simulink model "sampleModel187"  (R2021b)
settings: Solver=VariableStepAuto  StartTime=0.0  StopTime=10.0  RelTol=1e-3
undefined symbols (not defined in the file or in its folder): DiscIntNeverNeededParam, Newton, Raphson
libraries: simulink x10, slpidlib x1
settings Model: Creator=user  LastModifiedBy=user

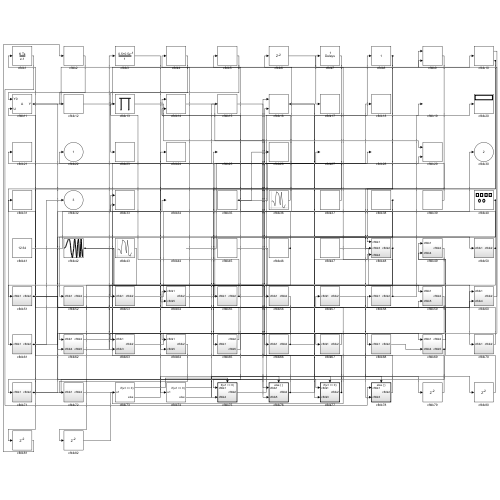
[thumbnail: Simulink's stored preview of the top-level diagram]
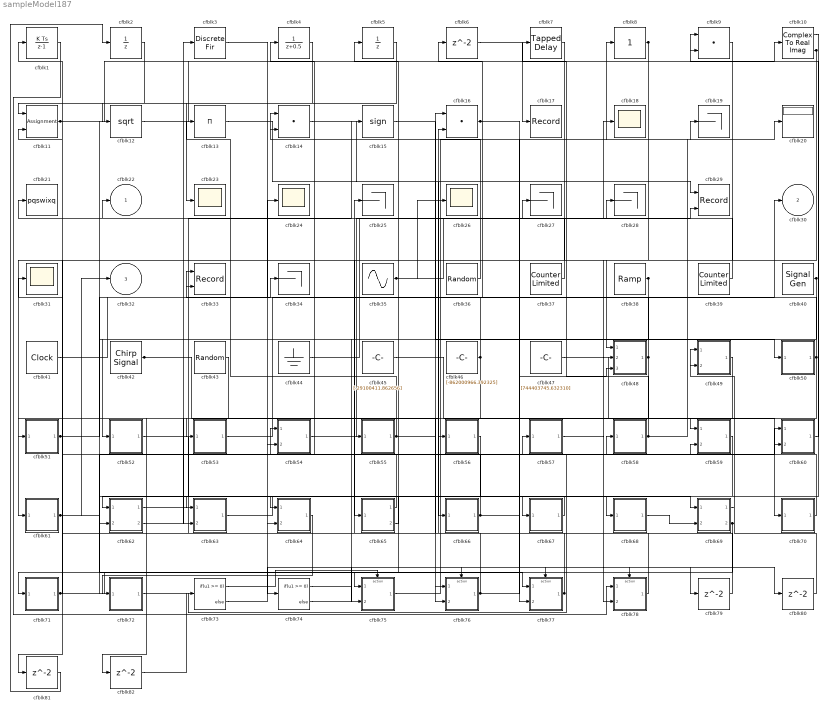
== system sampleModel187 ==
  cfblk1 : DiscreteIntegrator  ICPrevOutput=DiscIntNeverNeededParam  ICPrevScaledInput=DiscIntNeverNeededParam
  cfblk10 : ComplexToRealImag
  cfblk11 : Assignment  DiagnosticForDimensions=Warning  IndexOptions=Index vector (dialog)  Indices=1  OutputSizes=1
  cfblk12 : Sqrt  SaturateOnIntegerOverflow=on
  cfblk13 : Product  Inputs=*
  cfblk14 : DotProduct  InputSameDT=on  OutDataTypeStr=Inherit: Inherit via internal rule
  cfblk15 : Signum
  cfblk16 : DotProduct  InputSameDT=on  OutDataTypeStr=Inherit: Inherit via internal rule
  cfblk17 : Record  FileSettingsInternal="{\"entries\":[{\"content\":{\"excelSettings\":{\"content\":{},\"type\":\"Streamout.ExcelSettings\"}},\"type\":\"Streamout.FileSettingStorage\",\"uuid\":\"fc1a8ae5-f9e8-4fe5-bdf4-1e206a54b291\"}],\"packageUris\":[\"http://schema.mathworks.com/mf0/streamout_blocks/R2020a\"],\"version\":\"1.0\"}"  SignalsInternal="{\"entries\":[{\"content\":{\"signals\":[{\"content\":{\"blockPath\":[\"sampleModel187/cfblk17\"],\"channel\":[],\"dimensions\":[1],\"domain\":\"sampleModel187/cfblk17\",\"lineColor\":\"#d95319\",\"plots\":[1],\"port\":1,\"sid\":[\"\"],\"signalID\":7009,\"signalName\":\"cfblk6\"},\"type\":\"RecordBlkView.Signal\",\"uuid\":\"a0e15be2-1bcc-4cfc-9ff8-bd1e4d51e042\"}]},\"type\":\"RecordBlkView.InputSignals\",\"uuid\":\"3d8c80d8-74ea-49cf-8dca-ff953d23ae87\"}],\"packageUris\":[\"http://schema.mathworks.com/mf0/streamout_blocks/R2020a\"],\"version\":\"1.0\"}"  VisualizationBindings="{\"sparklinesplugin\":{\"info\":[{\"bindingParametersList\":[],\"subplotID\":1}]}}"
  cfblk{18,23..24,26,31} (5 alike) : Scope
  cfblk{19,25,27..28,34} (5 alike) : Terminator
  cfblk2 : UnitDelay  HasFrameUpgradeWarning=on
  cfblk20 : Display
  cfblk21 : ToWorkspace  VariableName=pqswixq  SaveFormat=Timeseries  SampleTime=-1
  cfblk29 : Record  FileSettingsInternal="{\"entries\":[{\"content\":{\"excelSettings\":{\"content\":{},\"type\":\"Streamout.ExcelSettings\"}},\"type\":\"Streamout.FileSettingStorage\",\"uuid\":\"442cfed6-b428-4296-b731-16461bc16b9e\"}],\"packageUris\":[\"http://schema.mathworks.com/mf0/streamout_blocks/R2020a\"],\"version\":\"1.0\"}"  Layout=[1 1]  SignalsInternal="{\"entries\":[{\"content\":{\"signals\":[{\"content\":{\"blockPath\":[\"sampleModel187/cfblk29\"],\"channel\":[],\"dimensions\":[1],\"domain\":\"sampleModel187/cfblk29\",\"lineColor\":\"#a2142f\",\"plots\":[1],\"port\":1,\"sid\":[\"\"],\"signalID\":7013,\"signalName\":\"cfblk14\"},\"type\":\"RecordBlkView.Signal\",\"uuid\":\"7f7e597a-58f6-4f39-b89b-6fa5513463cd\"},{\"content\":{\"blockPath\":[\"sampleModel187/cfblk29\"],\"channel\":[],\"dimensions\":[1],\"domain\":\"sampleModel187/cfblk29\",\"lineColor\":\"#139fff\",\"plots\":[1],\"port\":2,\"sid\":[\"\"],\"signalID\":7017,\"signalName\":\"cfblk35\"},\"type\":\"RecordBlkView.Signal\",\"uuid\":\"f445a410-3b6b-46a1-9c78-5c7b7ec1c4c9\"}]},\"type\":\"RecordBlkView.InputSignals\",\"uuid\":\"241168fc-4b68-43ee-8138-e2bf9d0c6355\"}],\"packageUris\":[\"http://schema.mathworks.com/mf0/streamout_blocks/R2020a\"],\"version\":\"1.0\"}"  VisualizationBindings="{\"xyplotplugin\":{\"info\":[{\"series\":[{\"bindingParametersList\":[{\"parameter\":\"X-Axis\",\"signalID\":7013,\"signalName\":\"cfblk14\"},{\"parameter\":\"Y-Axis\",\"signalID\":7017,\"signalName\":\"cfblk35\"}],\"seriesID\":40900}],\"subplotID\":1}]}}"  CompatibilityTag=XY
  cfblk3 : DiscreteFir  SampleTime=1
  cfblk33 : Record  FileSettingsInternal="{\"entries\":[{\"content\":{\"excelSettings\":{\"content\":{},\"type\":\"Streamout.ExcelSettings\"}},\"type\":\"Streamout.FileSettingStorage\",\"uuid\":\"6813dc0c-da85-4995-987b-cf181cce3f56\"}],\"packageUris\":[\"http://schema.mathworks.com/mf0/streamout_blocks/R2020a\"],\"version\":\"1.0\"}"  Layout=[1 1]  SignalsInternal="{\"entries\":[{\"content\":{\"signals\":[{\"content\":{\"blockPath\":[\"sampleModel187/cfblk33\"],\"channel\":[],\"dimensions\":[1],\"domain\":\"sampleModel187/cfblk33\",\"lineColor\":\"#a2142f\",\"plots\":[1],\"port\":1,\"sid\":[\"\"],\"signalID\":7021,\"signalName\":\"cfblk51\"},\"type\":\"RecordBlkView.Signal\",\"uuid\":\"0b49e028-e18d-4d9a-83a4-6c0870952cad\"},{\"content\":{\"blockPath\":[\"sampleModel187/cfblk33\"],\"channel\":[],\"dimensions\":[1],\"domain\":\"sampleModel187/cfblk33\",\"lineColor\":\"#139fff\",\"plots\":[1],\"port\":2,\"sid\":[\"\"],\"signalID\":7025,\"signalName\":\"cfblk46\"},\"type\":\"RecordBlkView.Signal\",\"uuid\":\"72cd62b7-a94f-45b4-8cbc-2f72f91e9fed\"}]},\"type\":\"RecordBlkView.InputSignals\",\"uuid\":\"c025e356-637a-424e-9c4b-b7d8cce8fa36\"}],\"packageUris\":[\"http://schema.mathworks.com/mf0/streamout_blocks/R2020a\"],\"version\":\"1.0\"}"  VisualizationBindings="{\"xyplotplugin\":{\"info\":[{\"series\":[{\"bindingParametersList\":[{\"parameter\":\"X-Axis\",\"signalID\":7021,\"signalName\":\"cfblk51\"},{\"parameter\":\"Y-Axis\",\"signalID\":7025,\"signalName\":\"cfblk46\"}],\"seriesID\":1856}],\"subplotID\":1}]}}"  CompatibilityTag=XY
  cfblk35 : Sin  Amplitude=[317053556.111391]  Bias=[742690337.513964]  SampleTime=0
  cfblk36 : RandomNumber  Mean=[77071.071490]  Variance=[36157.270666]  Seed=[984000208.000000]  SampleTime=0.1
  cfblk37 : simulink/Sources/Counter Limited  uplimit=[72.000000]  tsamp=-1
  cfblk38 : simulink/Sources/Ramp  slope=[-3760.220899]  start=[27.940516]  InitialOutput=[-463211.106441]
  cfblk39 : simulink/Sources/Counter Limited  uplimit=[234.000000]  tsamp=-1
  cfblk4 : DiscreteTransferFcn  SampleTime=1
  cfblk40 : SignalGenerator  WaveForm=sawtooth  Amplitude=[-571267794.185304]
  cfblk41 : DigitalClock
  cfblk42 : simulink/Sources/Chirp Signal  f1=[-681070782.822331]  T=[-12766538.982882]  f2=[-716220490.810942]
  cfblk43 : RandomNumber  Mean=[4117.333607]  Variance=[38168.376727]  Seed=[309807594.000000]  SampleTime=0.1
  cfblk44 : Ground
  cfblk45 : Constant  Value=[-29100411.862656]  SampleTime=1
  cfblk46 : Constant  Value=[-862000966.392325]  SampleTime=1
  cfblk47 : Constant  Value=[744403745.632310]  SampleTime=1
  cfblk48 : Subsystem
  cfblk49 : Subsystem
  cfblk5 : UnitDelay  HasFrameUpgradeWarning=on
  cfblk50 : Subsystem
  cfblk51 : Subsystem
  cfblk52 : Subsystem
  cfblk53 : Subsystem
  cfblk54 : Subsystem
  cfblk55 : Subsystem
  cfblk56 : Subsystem
  cfblk57 : Subsystem
  cfblk58 : Subsystem
  cfblk59 : Subsystem
  cfblk{6,79..82} (5 alike) : Delay  SampleTime=1
  cfblk60 : Subsystem
  cfblk61 : Subsystem
  cfblk62 : Subsystem
  cfblk63 : Subsystem
  cfblk64 : Subsystem
  cfblk65 : Subsystem
  cfblk66 : Subsystem
  cfblk67 : Subsystem
  cfblk68 : Subsystem
  cfblk69 : Subsystem
  cfblk7 : simulink/Discrete/Tapped Delay  vinit=0.0  samptime=-1  NumDelays=1  DelayOrder=Oldest  includeCurrent=off
  cfblk70 : Subsystem
  cfblk71 : Subsystem
  cfblk72 : Subsystem
  cfblk73 : If  IfExpression=u1 >= 0  SampleTime=1
  cfblk74 : If  IfExpression=u1 >= 0  SampleTime=1
  cfblk75 : Subsystem  TreatAsAtomicUnit=on
  cfblk76 : Subsystem  TreatAsAtomicUnit=on
  cfblk77 : Subsystem  TreatAsAtomicUnit=on
  cfblk78 : Subsystem  TreatAsAtomicUnit=on
  cfblk8 : simulink/Math Operations/Slider Gain  gain=1  low=0  high=2
  cfblk9 : DotProduct  InputSameDT=on  OutDataTypeStr=Inherit: Inherit via internal rule
  cfblk22 : Outport
  cfblk30 : Outport  Port=2
  cfblk32 : Outport  Port=3
  wires:
  cfblk39/1 -> cfblk22/1
  cfblk53/1(cfblk2) -> cfblk30/1
  cfblk54/1(cfblk2) -> cfblk28/1
  cfblk61/1(cfblk2) -> cfblk32/1, cfblk64/1(cfblk1)
  cfblk77/1(cfblk2) -> cfblk34/1, cfblk1/1
  cfblk75/1(cfblk2) -> cfblk8/1
  cfblk5/1 -> cfblk11/1
  cfblk70/1(cfblk2) -> cfblk58/1(cfblk1)
  cfblk72/1(cfblk2) -> cfblk57/1(cfblk1)
  cfblk14/1 -> cfblk29/1
  cfblk71/1(cfblk2) -> cfblk77/1(cfblk1), cfblk60/1(cfblk1), cfblk11/2
  cfblk78/1(cfblk2) -> cfblk25/1
  cfblk4/1 -> cfblk23/1
  cfblk76/1(cfblk2) -> cfblk16/2, cfblk48/3(cfblk4)
  cfblk15/1 -> cfblk50/1(cfblk1)
  cfblk35/1 -> cfblk29/2, cfblk26/1
  cfblk46/1 -> cfblk61/1(cfblk1), cfblk33/2
  cfblk62/1(cfblk2) -> cfblk15/1
  cfblk60/1(cfblk2) -> cfblk9/1
  cfblk12/1 -> cfblk10/1
  cfblk55/1(cfblk2) -> cfblk13/1, cfblk27/1
  cfblk7/1 -> cfblk51/1(cfblk1)
  cfblk9/1 -> cfblk65/1(cfblk1)
  cfblk59/1(cfblk2) -> cfblk75/1(cfblk1)
  cfblk48/1(cfblk2) -> cfblk6/1, cfblk53/1(cfblk1), cfblk72/1(cfblk1)
  cfblk1/1 -> cfblk78/1(cfblk1)
  cfblk11/1 -> cfblk9/2, cfblk76/2(cfblk5)
  cfblk41/1 -> cfblk24/1
  cfblk6/1 -> cfblk17/1
  cfblk2/1 -> cfblk12/1
  cfblk3/1 -> cfblk74/1
  cfblk44/1 -> cfblk18/1
  cfblk47/1 -> cfblk59/1(cfblk1)
  cfblk58/1(cfblk2) -> cfblk7/1, cfblk20/1
  cfblk37/1 -> cfblk21/1
  cfblk65/1(cfblk2) -> cfblk14/1
  cfblk42/1 -> cfblk66/1(cfblk1), cfblk76/1(cfblk1)
  cfblk10/1 -> cfblk67/1(cfblk1)
  cfblk40/1 -> cfblk52/1(cfblk1), cfblk62/2(cfblk4)
  cfblk10/2 -> cfblk48/1(cfblk1), cfblk81/1
  cfblk45/1 -> cfblk70/1(cfblk1)
  cfblk63/1(cfblk2) -> cfblk68/1(cfblk1)
  cfblk66/1(cfblk2) -> cfblk19/1, cfblk31/1
  cfblk16/1 -> cfblk48/2(cfblk3), cfblk80/1
  cfblk50/1(cfblk2) -> cfblk5/1, cfblk54/2(cfblk5)
  cfblk51/1(cfblk2) -> cfblk59/2(cfblk5), cfblk33/1, cfblk60/2(cfblk4)
  cfblk49/1(cfblk2) -> cfblk55/1(cfblk1)
  cfblk36/1 -> cfblk4/1
  cfblk67/1(cfblk2) -> cfblk63/1(cfblk1)
  cfblk13/1 -> cfblk56/1(cfblk1)
  cfblk8/1 -> cfblk78/2(cfblk3), cfblk64/2(cfblk5)
  cfblk38/1 -> cfblk75/2(cfblk4), cfblk77/2(cfblk3)
  cfblk56/1(cfblk2) -> cfblk62/1(cfblk1)
  cfblk62/2(cfblk5) -> cfblk3/1
  cfblk52/1(cfblk2) -> cfblk69/1(cfblk1)
  cfblk69/1(cfblk2) -> cfblk49/1(cfblk1)
  cfblk65/2(cfblk5) -> cfblk14/2
  cfblk43/1 -> cfblk63/2(cfblk3)
  cfblk69/2(cfblk5) -> cfblk71/1(cfblk1), cfblk54/1(cfblk1)
  cfblk68/1(cfblk2) -> cfblk69/2(cfblk4)
  cfblk73/1 -> cfblk75/Action
  cfblk73/2 -> cfblk76/Action
  cfblk74/1 -> cfblk77/Action
  cfblk74/2 -> cfblk78/Action
  cfblk57/1(cfblk2) -> cfblk79/1
  cfblk79/1 -> cfblk16/1
  cfblk80/1 -> cfblk49/2(cfblk4)
  cfblk81/1 -> cfblk2/1
  cfblk64/1(cfblk2) -> cfblk82/1
  cfblk82/1 -> cfblk73/1

== system sampleModel187/cfblk48 ==
  cfblk1 : Inport
  cfblk3 : Inport  Port=2
  cfblk4 : Inport  Port=3
  cfblk2 : Outport
  wires:
  cfblk3/1 -> cfblk2/1

== system sampleModel187/cfblk49 ==
  cfblk1 : Inport
  cfblk4 : Inport  Port=2
  cfblk3 : Constant  Value=[613731018.959351]  SampleTime=1
  cfblk2 : Outport
  wires:
  cfblk3/1 -> cfblk2/1

== system sampleModel187/cfblk50 ==
  cfblk1 : Inport
  cfblk3 : Product  Inputs=**
  cfblk2 : Outport
  wires:
  cfblk1/1 -> cfblk2/1, cfblk3/1, cfblk3/2

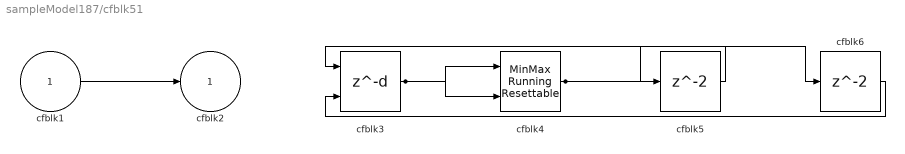
== system sampleModel187/cfblk51 ==
  cfblk1 : Inport
  cfblk3 : Delay  DelayLengthSource=Input port  SampleTime=1
      settings: InputPortMap=u0,p1
  cfblk4 : simulink/Math Operations/MinMax Running Resettable  Function=min  vinit=0.0
  cfblk5 : Delay  SampleTime=1
  cfblk6 : Delay  SampleTime=1
  cfblk2 : Outport
  wires:
  cfblk1/1 -> cfblk2/1
  cfblk3/1 -> cfblk4/1, cfblk4/2
  cfblk4/1 -> cfblk5/1, cfblk6/1
  cfblk5/1 -> cfblk3/1
  cfblk6/1 -> cfblk3/2

== system sampleModel187/cfblk52 ==
  cfblk1 : Inport
  cfblk3 : Trigonometry
  cfblk4 : simulink/Math Operations/Slider Gain  gain=1  low=0  high=2
  cfblk2 : Outport
  wires:
  cfblk1/1 -> cfblk4/1
  cfblk3/1 -> cfblk2/1
  cfblk4/1 -> cfblk3/1

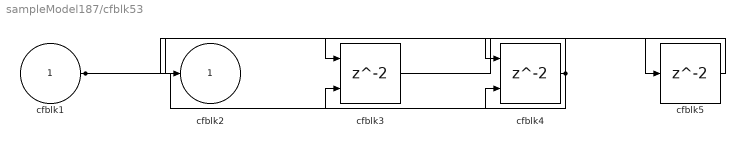
== system sampleModel187/cfblk53 ==
  cfblk1 : Inport
  cfblk3 : Delay  ShowEnablePort=on  SampleTime=1
      settings: InputPortMap=u0,e6
  cfblk4 : Delay  ShowEnablePort=on  SampleTime=1
      settings: InputPortMap=u0,e6
  cfblk5 : Delay  SampleTime=1
  cfblk2 : Outport
  wires:
  cfblk1/1 -> cfblk4/2, cfblk3/1
  cfblk4/1 -> cfblk2/1, cfblk3/2
  cfblk3/1 -> cfblk5/1
  cfblk5/1 -> cfblk4/1

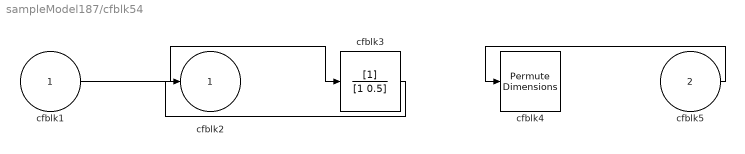
== system sampleModel187/cfblk54 ==
  cfblk1 : Inport
  cfblk5 : Inport  Port=2
  cfblk3 : DiscreteFilter  SampleTime=1
  cfblk4 : PermuteDimensions
  cfblk2 : Outport
  wires:
  cfblk5/1 -> cfblk4/1
  cfblk1/1 -> cfblk3/1
  cfblk3/1 -> cfblk2/1

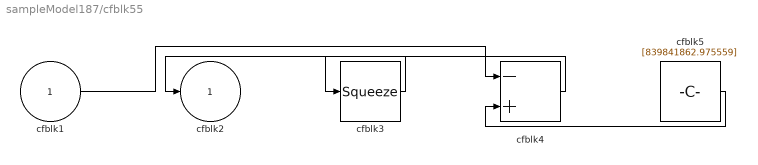
== system sampleModel187/cfblk55 ==
  cfblk1 : Inport
  cfblk3 : Squeeze
  cfblk4 : Sum  Inputs=-+
  cfblk5 : Constant  Value=[839841862.975559]  SampleTime=1
  cfblk2 : Outport
  wires:
  cfblk3/1 -> cfblk2/1
  cfblk1/1 -> cfblk4/1
  cfblk5/1 -> cfblk4/2
  cfblk4/1 -> cfblk3/1

== system sampleModel187/cfblk56 ==
  cfblk1 : Inport
  cfblk3 : Sum  Inputs=+-
  cfblk2 : Outport
  wires:
  cfblk1/1 -> cfblk3/1, cfblk3/2
  cfblk3/1 -> cfblk2/1

== system sampleModel187/cfblk57 ==
  cfblk1 : Inport
  cfblk3 : Constant  Value=[-506074840.334967]  SampleTime=1
  cfblk2 : Outport
  wires:
  cfblk3/1 -> cfblk2/1

== system sampleModel187/cfblk58 ==
  cfblk1 : Inport
  cfblk3 : Sqrt  Operator=rSqrt  AlgorithmType=Newton-Raphson  SaturateOnIntegerOverflow=on
  cfblk2 : Outport
  wires:
  cfblk1/1 -> cfblk3/1
  cfblk3/1 -> cfblk2/1

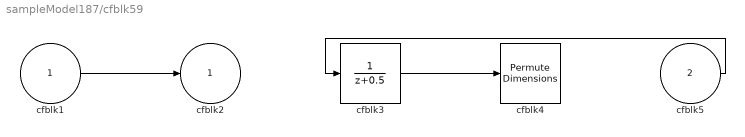
== system sampleModel187/cfblk59 ==
  cfblk1 : Inport
  cfblk5 : Inport  Port=2
  cfblk3 : DiscreteTransferFcn  SampleTime=1
  cfblk4 : PermuteDimensions
  cfblk2 : Outport
  wires:
  cfblk5/1 -> cfblk3/1
  cfblk3/1 -> cfblk4/1
  cfblk1/1 -> cfblk2/1

== system sampleModel187/cfblk60 ==
  cfblk1 : Inport
  cfblk4 : Inport  Port=2
  cfblk3 : Abs
  cfblk2 : Outport
  wires:
  cfblk4/1 -> cfblk3/1
  cfblk1/1 -> cfblk2/1

== system sampleModel187/cfblk61 ==
  cfblk1 : Inport
  cfblk3 : slpidlib/PID Controller  Controller=PID  Form=Parallel  TimeDomain=Discrete-time  UseExternalTs=off  SampleTime=1  IntegratorMethod=Forward Euler  FilterMethod=Forward Euler  ControllerParametersSource=internal  P=1  I=1  D=0  UseFilter=on  N=100  TunerSelectOption=Transfer Function Based (PID Tuner App)  InitialConditionSource=internal  InitialConditionForIntegrator=0  InitialConditionForFilter=0  DifferentiatorICPrevScaledInput=0  ExternalReset=none  TrackingMode=off  Kt=1  LimitOutput=off  SatLimitsSource=internal  UpperSaturationLimit=inf  LowerSaturationLimit=-inf  LinearizeAsGain=off  AntiWindupMode=none  Kb=1  POutMin=[]  POutMax=[]  IOutMin=[]  IOutMax=[]  DOutMin=[]  DOutMax=[]  NOutMin=[]  NOutMax=[]  SumOutMin=[]  SumOutMax=[]  SaturationOutMin=[]  SaturationOutMax=[]  PParamMin=[]  PParamMax=[]  IParamMin=[]  IParamMax=[]  DParamMin=[]  DParamMax=[]  NParamMin=[]  NParamMax=[]  KbParamMin=[]  KbParamMax=[]  KtParamMin=[]  KtParamMax=[]  KbOutMin=[]  KbOutMax=[]  KtOutMin=[]  KtOutMax=[]  IntegratorOutMin=[]  IntegratorOutMax=[]  FilterOutMin=[]  FilterOutMax=[]  SumI1OutMin=[]  SumI1OutMax=[]  SumI2OutMin=[]  SumI2OutMax=[]  SumI3OutMin=[]  SumI3OutMax=[]  SumI4OutMin=[]  SumI4OutMax=[]  SumDOutMin=[]  SumDOutMax=[]  DifferentiatorOutMin=[]  DifferentiatorOutMax=[]  FilterDiffOutCoefMin=[]  FilterDiffOutCoefMax=[]  ReciprocalOutMin=[]  ReciprocalOutMax=[]  SumDenOutMin=[]  SumDenOutMax=[]  SumNumOutMin=[]  SumNumOutMax=[]  DivideOutMin=[]  DivideOutMax=[]  UdiffTsProdOutMin=[]  UdiffTsProdOutMax=[]  NTsProdOutMin=[]  NTsProdOutMax=[]  UintegralTsProdOutMin=[]  UintegralTsProdOutMax=[]  UngainTsProdOutMin=[]  UngainTsProdOutMax=[]  IntegratorContinuousStateAttributes=''  IntegratorStateMustResolveToSignalObject=off  IntegratorRTWStateStorageClass=Auto  FilterContinuousStateAttributes=''  FilterStateMustResolveToSignalObject=off  FilterRTWStateStorageClass=Auto  ParallelPVariant=InternalParameters  IdealPVariant=Disabled  IVariant=InternalParameters  DVariant=InternalParameters  IntegratorVariant=Discrete  SatVariant=Disabled  AWVariant=Passthrough  PCopyVariant=Disabled  TRVariant=Disabled  FdbkBlocksVariant=Forward  IdealPFdbkVariant=Disabled  SatFdbkVariant=Disabled  DerivativeFilterVariant=ForwardEulerFilter  NVariant=InternalParameters  NCopyVariant=Disabled  FilterICVariant=InternalICsFilter  IntegratorICVariant=InternalICs  ExternalResetVariant=Disabled  TRSumVariant=Passthrough  SumFdbkVariant=Disabled  SumVariant=Sum_PID  TsampFilterVariant=InternalTs  TsampNgainVariant=Passthrough  TsampIntegralVariant=Passthrough  ExternalSaturationOutDataTypeStr=Inherit: Same as second input
  cfblk4 : ComplexToMagnitudeAngle
  cfblk2 : Outport
  wires:
  cfblk4/1 -> cfblk3/1
  cfblk3/1 -> cfblk2/1
  cfblk1/1 -> cfblk4/1

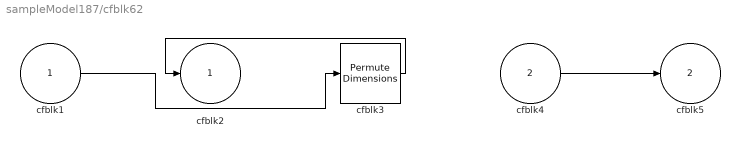
== system sampleModel187/cfblk62 ==
  cfblk1 : Inport
  cfblk4 : Inport  Port=2
  cfblk3 : PermuteDimensions
  cfblk2 : Outport
  cfblk5 : Outport  Port=2
  wires:
  cfblk3/1 -> cfblk2/1
  cfblk1/1 -> cfblk3/1
  cfblk4/1 -> cfblk5/1

== system sampleModel187/cfblk63 ==
  cfblk1 : Inport
  cfblk3 : Inport  Port=2
  cfblk2 : Outport
  wires:
  cfblk3/1 -> cfblk2/1

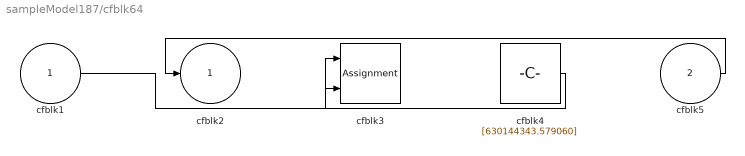
== system sampleModel187/cfblk64 ==
  cfblk1 : Inport
  cfblk5 : Inport  Port=2
  cfblk3 : Assignment  DiagnosticForDimensions=Warning  IndexOptions=Index vector (dialog)  Indices=1  OutputSizes=1
  cfblk4 : Constant  Value=[630144343.579060]  SampleTime=1
  cfblk2 : Outport
  wires:
  cfblk5/1 -> cfblk2/1
  cfblk1/1 -> cfblk3/1
  cfblk4/1 -> cfblk3/2

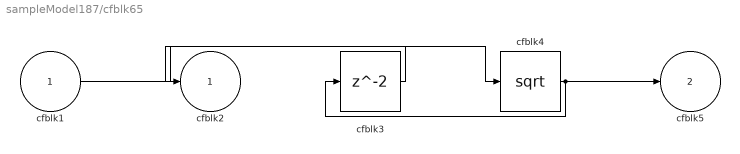
== system sampleModel187/cfblk65 ==
  cfblk1 : Inport
  cfblk3 : Delay  SampleTime=1
  cfblk4 : Sqrt  SaturateOnIntegerOverflow=on
  cfblk2 : Outport
  cfblk5 : Outport  Port=2
  wires:
  cfblk1/1 -> cfblk4/1
  cfblk4/1 -> cfblk3/1, cfblk5/1
  cfblk3/1 -> cfblk2/1

== system sampleModel187/cfblk66 ==
  cfblk1 : Inport
  cfblk3 : DiscreteFilter  SampleTime=1
  cfblk2 : Outport
  wires:
  cfblk1/1 -> cfblk2/1, cfblk3/1

== system sampleModel187/cfblk67 ==
  cfblk1 : Inport
  cfblk3 : Sum  Inputs=|++
  cfblk2 : Outport
  wires:
  cfblk1/1 -> cfblk3/1, cfblk3/2
  cfblk3/1 -> cfblk2/1

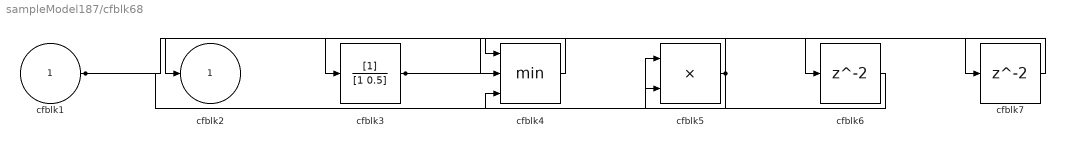
== system sampleModel187/cfblk68 ==
  cfblk1 : Inport
  cfblk3 : DiscreteFilter  SampleTime=1
  cfblk4 : MinMax  Inputs=3
  cfblk5 : Product  Inputs=**
  cfblk6 : Delay  SampleTime=1
  cfblk7 : Delay  SampleTime=1
  cfblk2 : Outport
  wires:
  cfblk5/1 -> cfblk2/1, cfblk4/3
  cfblk1/1 -> cfblk5/1, cfblk4/2
  cfblk3/1 -> cfblk6/1, cfblk7/1
  cfblk4/1 -> cfblk3/1
  cfblk6/1 -> cfblk5/2
  cfblk7/1 -> cfblk4/1

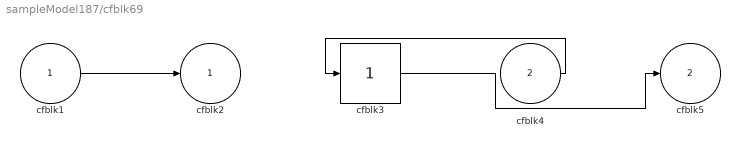
== system sampleModel187/cfblk69 ==
  cfblk1 : Inport
  cfblk4 : Inport  Port=2
  cfblk3 : simulink/Math Operations/Slider Gain  gain=1  low=0  high=2
  cfblk2 : Outport
  cfblk5 : Outport  Port=2
  wires:
  cfblk4/1 -> cfblk3/1
  cfblk1/1 -> cfblk2/1
  cfblk3/1 -> cfblk5/1

== system sampleModel187/cfblk70 ==
  cfblk1 : Inport
  cfblk3 : Delay  SampleTime=1
  cfblk4 : Delay  DelayLengthSource=Input port  SampleTime=1
      settings: InputPortMap=u0,p1
  cfblk5 : Delay  SampleTime=1
  cfblk2 : Outport
  wires:
  cfblk1/1 -> cfblk4/1
  cfblk3/1 -> cfblk2/1, cfblk5/1
  cfblk4/1 -> cfblk3/1
  cfblk5/1 -> cfblk4/2

== system sampleModel187/cfblk71 ==
  cfblk1 : Inport
  cfblk3 : simulink/Discrete/Transfer Fcn First Order  PoleZ=0.95  ICPrevOutput=0.0  DoSatur=off
  cfblk4 : UnitDelay  HasFrameUpgradeWarning=on
  cfblk5 : Abs
  cfblk2 : Outport
  wires:
  cfblk3/1 -> cfblk5/1
  cfblk5/1 -> cfblk4/1
  cfblk4/1 -> cfblk2/1
  cfblk1/1 -> cfblk3/1

== system sampleModel187/cfblk72 ==
  cfblk1 : Inport
  cfblk3 : DiscreteFilter  SampleTime=1
  cfblk2 : Outport
  wires:
  cfblk1/1 -> cfblk2/1, cfblk3/1

== system sampleModel187/cfblk75 ==
  cfblk1 : Inport
  cfblk4 : Inport  Port=2
  Action Port : ActionPort  ActionPortLabel=if(u1 >= 0)
  cfblk3 : DiscreteZeroPole  Poles=[0 0.5]  Gain=1  SampleTime=-1
  cfblk2 : Outport
  wires:
  cfblk1/1 -> cfblk3/1
  cfblk3/1 -> cfblk2/1

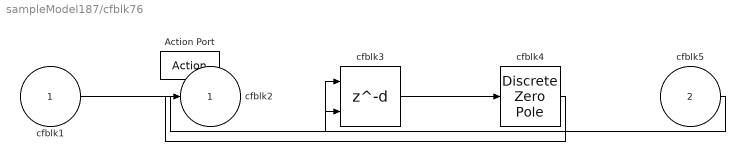
== system sampleModel187/cfblk76 ==
  cfblk1 : Inport
  cfblk5 : Inport  Port=2
  Action Port : ActionPort  ActionPortLabel=else
  cfblk3 : Delay  DelayLengthSource=Input port
      settings: InputPortMap=u0,p1
  cfblk4 : DiscreteZeroPole  Poles=[0 0.5]  Gain=1  SampleTime=-1
  cfblk2 : Outport
  wires:
  cfblk1/1 -> cfblk3/1
  cfblk4/1 -> cfblk2/1
  cfblk3/1 -> cfblk4/1
  cfblk5/1 -> cfblk3/2

== system sampleModel187/cfblk77 ==
  cfblk1 : Inport
  cfblk3 : Inport  Port=2
  Action Port : ActionPort  ActionPortLabel=if(u1 >= 0)
  cfblk2 : Outport
  wires:
  cfblk1/1 -> cfblk2/1

== system sampleModel187/cfblk78 ==
  cfblk1 : Inport
  cfblk3 : Inport  Port=2
  Action Port : ActionPort  ActionPortLabel=else
  cfblk2 : Outport
  wires:
  cfblk1/1 -> cfblk2/1
